simulink model "Perfect_nav"  (R2018b)
settings: configuration reference "Configuration" (kept outside this file)
model workspace (MATLAB code in the model file):
  | CON = Simulink.Parameter;
  | CON.DataType = 'Bus: Bus_CON';
  | CON.Value = Simulink.Bus.createMATLABStruct('Bus_CON');
settings Model: ParameterArgumentNames=CON  OrderedModelArguments=off  Creator=Ethan  LastModifiedBy=Ethan
settings ConfigSetRef: SourceLocation=Base Workspace

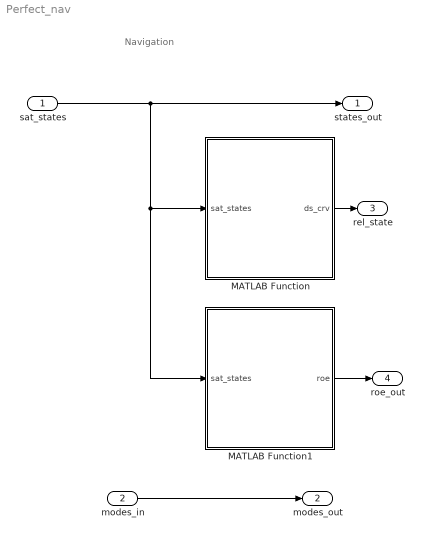
== system Perfect_nav ==
  note: Navigation
  sat_states : Inport  OutDataTypeStr=Bus: Bus_outputs
  modes_in : Inport  Port=2  OutDataTypeStr=Bus: Bus_modes
  MATLAB Function : MATLAB Function  TreatAsAtomicUnit=on
  MATLAB Function1 : MATLAB Function  TreatAsAtomicUnit=on
  states_out : Outport  OutDataTypeStr=Bus: Bus_outputs
  modes_out : Outport  Port=2  OutDataTypeStr=Bus: Bus_modes
  rel_state : Outport  Port=3
  roe_out : Outport  Port=4  OutDataTypeStr=Bus: Bus_roe
  wires:
  modes_in/1 -> modes_out/1
  sat_states/1 -> MATLAB Function1/1(sat_states), MATLAB Function/1(sat_states), states_out/1
  MATLAB Function/1(ds_crv) -> rel_state/1
  MATLAB Function1/1(roe) -> roe_out/1

== matlab function Perfect_nav/MATLAB Function1 ==
  data: sat_states input; roe output Bus: Bus_roe; CON parameter
function roe  = i2roe(sat_states, CON)
persistent da_prev

chief = sat_states.NXS_out;
deputy = sat_states.astro_out;
[ac,ec,ic,oc,wc,~, uc] = rvECI2oe_rad(chief.r_i, chief.v_i, CON.mu);
[ad,ed,id,od,wd,~, ud] = rvECI2oe_rad(deputy.r_i, deputy.v_i, CON.mu);

if isempty(da_prev)
    da_prev = (ad - ac) / ac;
end

% 
moe_c = osc2mean([ac,ec,ic,oc,wc, uc], CON.Re, CON.J2);
moe_d = osc2mean([ad,ed,id,od,wd, ud] , CON.Re, CON.J2);
% 
% ac = moe_c(1);
% ec = moe_c(2);
% ic = moe_c(3);
% oc = moe_c(4);
% wc = moe_c(5);
% uc = moe_c(6);
% 
% ad = moe_d(1);
% ed = moe_d(2);
% id = moe_d(3);
% od = moe_d(4);
% wd = moe_d(5);
% ud = moe_d(6);

% roe.adot =((ad - ac) / ac - da_prev) / CON.computer_dt;
% roe.da = (ad - ac) / ac;
% roe.dL = (ud - uc) + (od - oc) * cos(ic);
% roe.dex = ed * cos(wd) - ec * cos(wc);
% roe.dey = ed * sin(wd) - ec * sin(wc);
% roe.dix = id - ic;
% roe.diy = (od - oc) * sin(ic);

roetemp = oe2roe(moe_c, moe_d, 1);

roe.adot = -4.5075e-10;
roe.da = roetemp(1);
roe.dL = roetemp(2);
roe.dex = roetemp(3);
roe.dey = roetemp(4);
roe.dix = roetemp(5);
roe.diy = roetemp(6);
da_prev = roe.da;
end

== matlab function Perfect_nav/MATLAB Function ==
  data: sat_states input; ds_crv output
function ds_crv  = i2relRTN(sat_states)

chief = sat_states.NXS_out;
deputy = sat_states.astro_out;

[rHill,vHill] = ECI2Hill_Vectorized(chief.r_i,chief.v_i,deputy.r_i,deputy.v_i);
ds_crv = [rHill;vHill];
end
